simulink model "mcb_microchip_pmsm_autotuner_SAME70"  (R2023a)
settings: Solver=FixedStepDiscrete  StartTime=0.0  StopTime=30  RelTol=1e-3  EnableMultiTasking=on
InitFcn:
  | mcb_microchip_pmsm_autotuner_SAME70_data;
values from neighbouring files (symbols this model uses):
  PU_System = mcb_SetPUSystem(pmsm,inverter)    [mcb_microchip_pmsm_autotuner_SAME70_data.m]
  Ts = T_pwm    (= 5e-05)    [mcb_microchip_pmsm_autotuner_SAME70_data.m]
  Ts_motor = T_pwm/2    (= 2.5e-05)    [mcb_microchip_pmsm_autotuner_SAME70_data.m]
  Ts_simulink = T_pwm/2    (= 2.5e-05)    [mcb_microchip_pmsm_autotuner_SAME70_data.m]
  Ts_speed = 2 * Ts    (= 0.0001)    [mcb_microchip_pmsm_autotuner_SAME70_data.m]
undefined symbols (not defined in the file or in its folder): A24, AD10, AD7, inverter, LQFP144, MaxPer, ms, ns, PA0, PA1, PA10, PA11, PA12, PA13, PA16, PA18, PA9, PB0, PD18, PD19, PD24, PD25, PD26, PI_params, Pin, pmsm, Resol, SAME70Q21B, target, Timer, Unsigned
libraries: simulink x13, MCHP_Blockset x13, mcbcontrolslib x7, slpidlib x3, mcbpositiondecoderlib x3, svdutilitieslib x3, mcbplantlib x1, autolibpmsmexterior x1, focautotunershared x1
(part 4 of 4)

== system mcb_microchip_pmsm_autotuner_SAME70/Microcontroller/Input Scaling/Variant Subsystem/Automatic offset calibration ==
  Mode : Inport
  Iab_ADC : Inport  Port=2
  Add : Sum  Inputs=-+  RndMeth=Simplest  OutDataTypeStr=Inherit: Same as first input
  Compare To Constant : simulink/Logic and Bit Operations/Compare To Constant  relop=<  const=1  OutDataTypeStr=boolean
  Data Type Conversion : DataTypeConversion  OutDataTypeStr=int32  ConvertRealWorld=Stored Integer (SI)  RndMeth=Simplest  SaturateOnIntegerOverflow=off
  Enabled Subsystem : Subsystem  TreatAsAtomicUnit=on
  Gain : Gain  Gain=inverter.AmpPerCount  OutDataTypeStr=dataType  RndMeth=Simplest
  Iab : Outport
  wires:
  Data Type Conversion/1 -> Add/2, Enabled Subsystem/1(In1)
  Gain/1 -> Iab/1
  Enabled Subsystem/1(Out1) -> Add/1
  Add/1 -> Gain/1
  Compare To Constant/1 -> Enabled Subsystem/Enable
  Mode/1 -> Compare To Constant/1
  Iab_ADC/1 -> Data Type Conversion/1

== system mcb_microchip_pmsm_autotuner_SAME70/Microcontroller/Input Scaling/Variant Subsystem/Offser via parameter ==
  Mode : Inport
  Iab_ADC : Inport  Port=2
  Add : Sum  Inputs=-+  RndMeth=Simplest  OutDataTypeStr=Inherit: Same as first input
  Constant : Constant  Value=[inverter.CtSensAOffset inverter.CtSensBOffset]  OutDataTypeStr=Inherit: Inherit via back propagation
  Gain : Gain  Gain=inverter.AmpPerCount  OutDataTypeStr=dataType  RndMeth=Simplest
  Terminator : Terminator
  Iab : Outport
  wires:
  Gain/1 -> Iab/1
  Iab_ADC/1 -> Add/2
  Add/1 -> Gain/1
  Constant/1 -> Add/1
  Mode/1 -> Terminator/1

== system mcb_microchip_pmsm_autotuner_SAME70/Microcontroller/Output PWM Drivers/Sim/Subsystem ==
  PWM_In : Inport
  Constant : Constant  Value=0.5  OutDataTypeStr=dataType
  Gain : Gain  Gain=0.5  OutDataTypeStr=Inherit: Same as input
  Sum : Sum  Inputs=|++
  PWM_Duty_Cycles : Outport
  wires:
  Gain/1 -> Sum/1
  Constant/1 -> Sum/2
  PWM_In/1 -> Gain/1
  Sum/1 -> PWM_Duty_Cycles/1  "PWM_Duty_Cycles"

== system mcb_microchip_pmsm_autotuner_SAME70/Microcontroller/SCI In Abstraction/Variant Subsystem/Codegen ==
  SCI_Data : Inport
  Mode : Inport  Port=2
  AND : Logic  IconShape=distinctive  AllPortsSameDT=off  OutDataTypeStr=boolean
  Bus Creator : BusCreator  Inputs=4
  Compare To Constant : simulink/Logic and Bit Operations/Compare To Constant  relop=>=  const=2  OutDataTypeStr=boolean
  Data Type Conversion : DataTypeConversion  OutDataTypeStr=boolean  RndMeth=Simplest  SaturateOnIntegerOverflow=off
  Subsystem : Subsystem
  ConfigAndCommand : Outport
  DebugSel : Outport  Port=2
  wires:
  Bus Creator/1 -> ConfigAndCommand/1
  AND/1 -> Bus Creator/1  "Enable"
  Subsystem/1(Enable) -> AND/2
  Subsystem/2(AutoTuneEn) -> Data Type Conversion/1
  Subsystem/3(SpeedRef) -> Bus Creator/3  "SpeedRef"
  Subsystem/5(DebugSel) -> DebugSel/1
  Compare To Constant/1 -> AND/1
  Mode/1 -> Compare To Constant/1
  Subsystem/4(ResetPIParams) -> Bus Creator/4  "ResetPIGains"
  SCI_Data/1 -> Subsystem/1(SCI_Data)
  Data Type Conversion/1 -> Bus Creator/2  "AutoTuneEn"

== system mcb_microchip_pmsm_autotuner_SAME70/Microcontroller/SCI In Abstraction/Variant Subsystem/Sim ==
  SCI_Data : Inport
  Mode : Inport  Port=2
  AND : Logic  IconShape=distinctive  AllPortsSameDT=off  OutDataTypeStr=boolean
  Bus Creator : BusCreator  Inputs=4
  Compare To Constant : simulink/Logic and Bit Operations/Compare To Constant  relop=>=  const=2  OutDataTypeStr=boolean
  Constant : Constant  Value=1000  OutDataTypeStr=dataType  SampleTime=Ts
  Constant1 : Constant  OutDataTypeStr=uint8
  Constant2 : Constant  Value=0  OutDataTypeStr=boolean  SampleTime=Ts
  Data Type Conversion : DataTypeConversion  OutDataTypeStr=boolean  RndMeth=Simplest  SaturateOnIntegerOverflow=off
  Step : Step  Time=29  Before=1  After=0  SampleTime=Ts
  Step1 : Step  Time=4  SampleTime=Ts
  Terminator : Terminator
  ConfigAndCommand : Outport
  DebugSel : Outport  Port=2
  wires:
  SCI_Data/1 -> Terminator/1
  Mode/1 -> Compare To Constant/1
  Compare To Constant/1 -> AND/1
  Step/1 -> AND/2
  Bus Creator/1 -> ConfigAndCommand/1
  AND/1 -> Bus Creator/1  "Enable"
  Step1/1 -> Data Type Conversion/1
  Constant/1 -> Bus Creator/3  "SpeedRef"
  Constant1/1 -> DebugSel/1
  Constant2/1 -> Bus Creator/4  "ResetPIGains"
  Data Type Conversion/1 -> Bus Creator/2  "AutoTuneEn"

== system mcb_microchip_pmsm_autotuner_SAME70/Microcontroller/SCI_Rx/CodeGen/Subsystem ==
  In1 : Inport
  Enable1 : EnablePort
  Data : Outport
  wires:
  In1/1 -> Data/1

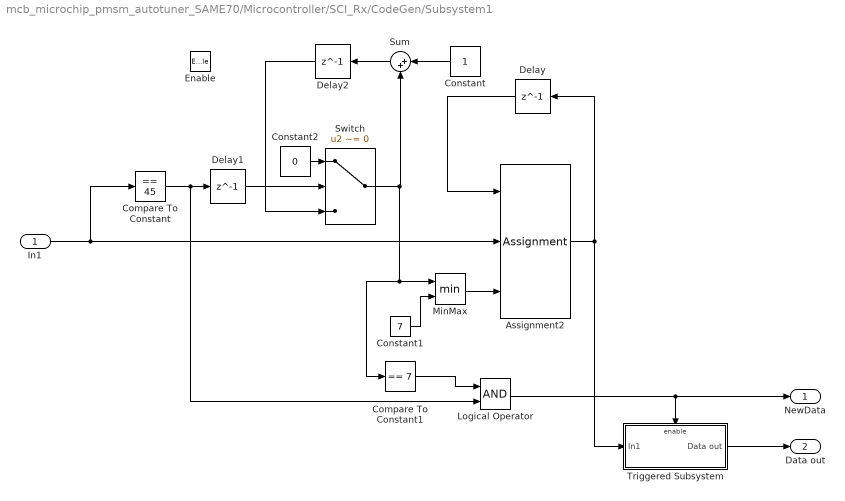
== system mcb_microchip_pmsm_autotuner_SAME70/Microcontroller/SCI_Rx/CodeGen/Subsystem1 ==
  In1 : Inport
  Enable : EnablePort
  Assignment2 : Assignment  IndexMode=Zero-based  DiagnosticForDimensions=Warning  IndexOptions=Starting index (port)  Indices=1  OutputSizes=1
  Compare To Constant : simulink/Logic and Bit Operations/Compare To Constant  relop===  const=45  OutDataTypeStr=boolean
  Compare To Constant1 : simulink/Logic and Bit Operations/Compare To Constant  relop===  const=7  OutDataTypeStr=boolean
  Constant : Constant  OutDataTypeStr=uint16  SampleTime=-1
  Constant1 : Constant  Value=7  OutDataTypeStr=uint16  SampleTime=-1
  Constant2 : Constant  Value=0  OutDataTypeStr=uint16  SampleTime=-1
  Delay : Delay  DelayLength=1  InitialCondition=[0 0 0 0 0 0 0 0]
  Delay1 : Delay  DelayLength=1  InitialCondition=0
  Delay2 : Delay  DelayLength=1  InitialCondition=0
  Logical Operator : Logic  AllPortsSameDT=off  OutDataTypeStr=boolean
  MinMax : MinMax  Inputs=2
  Sum : Sum  Inputs=|++
  Switch : Switch  Criteria=u2 ~= 0  SaturateOnIntegerOverflow=off  InputSameDT=off
  Triggered Subsystem : Subsystem  TreatAsAtomicUnit=on
  NewData : Outport  OutputWhenDisabled=reset  InitialOutput=0
  Data out : Outport  Port=2
  wires:
  Logical Operator/1 -> Triggered Subsystem/Enable, NewData/1
  Constant2/1 -> Switch/1
  Delay1/1 -> Switch/2
  Switch/1 -> MinMax/1, Compare To Constant1/1, Sum/2
  Sum/1 -> Delay2/1
  MinMax/1 -> Assignment2/3
  Constant1/1 -> MinMax/2
  Constant/1 -> Sum/1
  In1/1 -> Assignment2/2, Compare To Constant/1
  Compare To Constant1/1 -> Logical Operator/1
  Compare To Constant/1 -> Delay1/1, Logical Operator/2
  Delay2/1 -> Switch/3
  Delay/1 -> Assignment2/1
  Assignment2/1 -> Delay/1, Triggered Subsystem/1(In1)
  Triggered Subsystem/1(Data out) -> Data out/1

== system mcb_microchip_pmsm_autotuner_SAME70/Microcontroller/SCI_Tx/Codegen/Data ==
  Data : Inport
  Action Port : ActionPort  ActionPortLabel=else
  UART Tx : MCHP_Blockset/BUS UART/UART Tx  UART_REF=UART 0  ORDERING=None  AllOrNothing=off  SampleTime=-1  MCHP_MASTERLINK=mcb_microchip_pmsm_autotuner_SAME70/Microcontroller/Configurations/Microchip Master  NSend_Input=off  UART_String=off  NSend_Output=off
      settings: SourceProductName=MPLAB Device Blocks for Simulink
  wires:
  Data/1 -> UART Tx/1

== system mcb_microchip_pmsm_autotuner_SAME70/Microcontroller/SCI_Tx/Codegen/End ==
  Data : Inport
  Action Port : ActionPort  ActionPortLabel=elseif(u1 == single(target.SerialFrameSize-1))
  Mux : Mux  Inputs=2
  Start : Constant  Value=hex2dec('45')  OutDataTypeStr=uint8
  UART Tx : MCHP_Blockset/BUS UART/UART Tx  UART_REF=UART 0  ORDERING=None  AllOrNothing=off  SampleTime=-1  MCHP_MASTERLINK=mcb_microchip_pmsm_autotuner_SAME70/Microcontroller/Configurations/Microchip Master  NSend_Input=off  UART_String=off  NSend_Output=off
      settings: SourceProductName=MPLAB Device Blocks for Simulink
  wires:
  Start/1 -> Mux/2
  Data/1 -> Mux/1
  Mux/1 -> UART Tx/1

== system mcb_microchip_pmsm_autotuner_SAME70/Microcontroller/SCI_Tx/Codegen/Start ==
  Data : Inport
  Action Port : ActionPort  ActionPortLabel=if(u1 == 0)
  End : Constant  Value=hex2dec('53')  OutDataTypeStr=uint8
  Mux : Mux  Inputs=2
  UART Tx : MCHP_Blockset/BUS UART/UART Tx  UART_REF=UART 0  ORDERING=None  AllOrNothing=off  SampleTime=-1  MCHP_MASTERLINK=mcb_microchip_pmsm_autotuner_SAME70/Microcontroller/Configurations/Microchip Master  NSend_Input=off  UART_String=off  NSend_Output=off
      settings: SourceProductName=MPLAB Device Blocks for Simulink
  wires:
  End/1 -> Mux/1
  Data/1 -> Mux/2
  Mux/1 -> UART Tx/1

== system mcb_microchip_pmsm_autotuner_SAME70/Inverter and Motor/Inverter and Motor/Sim/Motor/Inverter ==
  Duty_abc : Inport
  Average-Value Inverter : mcbplantlib/Average-Value Inverter
  Constant2 : Constant  Value=inverter.V_dc  OutDataTypeStr=single  SampleTime=-1
  Data Type Conversion1 : DataTypeConversion  OutDataTypeStr=single  RndMeth=Simplest  SaturateOnIntegerOverflow=off
  Vabc : Outport
  wires:
  Constant2/1 -> Average-Value Inverter/2
  Duty_abc/1 -> Data Type Conversion1/1
  Average-Value Inverter/1 -> Vabc/1
  Data Type Conversion1/1 -> Average-Value Inverter/1

== system mcb_microchip_pmsm_autotuner_SAME70/Inverter and Motor/Inverter and Motor/Sim/Motor/Load_Profile (Torque) ==
  Data Type Conversion : DataTypeConversion  OutDataTypeStr=single  SaturateOnIntegerOverflow=off  RndMeth=Floor
  IIR Filter : mcbcontrolslib/IIR Filter  VariantControl=Low Pass Filter  VariantSelect=Low-pass  Filter_constant=0.0001  advancedSettings=off  Ts=50e-6  cutOff_freq=0.31834
  T_load : Step  Time=3  After=0  SampleTime=Ts_simulink
  Load_Trq : Outport  VectorParamsAs1DForOutWhenUnconnected=off
  wires:
  Data Type Conversion/1 -> IIR Filter/1
  IIR Filter/1 -> Load_Trq/1
  T_load/1 -> Data Type Conversion/1

== system mcb_microchip_pmsm_autotuner_SAME70/Microcontroller/Application/Current Control/Current_Controllers/PI_Controller_Id ==
  I_ref : Inport
  I_fb : Inport  Port=2
  En : Inport  Port=3
  PIParams : Inport  Port=4
  Bus Selector : BusSelector  OutputSignals=KpId,KiId
  Discrete PI Controller with anti-windup & reset : slpidlib/PID Controller  Controller=PI  Form=Parallel  TimeDomain=Discrete-time  UseExternalTs=off  SampleTime=-1  IntegratorMethod=Forward Euler  FilterMethod=Forward Euler  ControllerParametersSource=external  P=1  I=1  UseKiTs=on  D=0  N=100  UseFilter=on  TunerSelectOption=Transfer Function Based (PID Tuner App)  InitialConditionSource=external  InitialConditionForIntegrator=0  InitialConditionForFilter=0  DifferentiatorICPrevScaledInput=0  ExternalReset=level  TrackingMode=off  Kt=1  LimitOutput=on  SatLimitsSource=internal  UpperSaturationLimit=1  LowerSaturationLimit=-1  LinearizeAsGain=on  AntiWindupMode=clamping  Kb=1  LimitIntegrator=off  UpperIntegratorSaturationLimit=inf  LowerIntegratorSaturationLimit=-inf  RndMeth=Simplest  POutMin=[]  POutMax=[]  IOutMin=[]  IOutMax=[]  DOutMin=[]  DOutMax=[]  NOutMin=[]  NOutMax=[]  SumOutMin=[]  SumOutMax=[]  SaturationOutDataTypeStr=Inherit: Inherit via back propagation  SaturationOutMin=[]  SaturationOutMax=[]  PParamMin=[]  PParamMax=[]  IParamMin=[]  IParamMax=[]  DParamMin=[]  DParamMax=[]  NParamMin=[]  NParamMax=[]  KbParamMin=[]  KbParamMax=[]  KtParamMin=[]  KtParamMax=[]  KbOutMin=[]  KbOutMax=[]  KtOutMin=[]  KtOutMax=[]  IntegratorOutMin=[]  IntegratorOutMax=[]  FilterOutMin=[]  FilterOutMax=[]  SumI1OutMin=[]  SumI1OutMax=[]  SumI2OutMin=[]  SumI2OutMax=[]  SumI3OutMin=[]  SumI3OutMax=[]  SumI4OutMin=[]  SumI4OutMax=[]  SumDOutMin=[]  SumDOutMax=[]  DifferentiatorOutMin=[]  DifferentiatorOutMax=[]  FilterDiffOutCoefMin=[]  FilterDiffOutCoefMax=[]  ReciprocalOutMin=[]  ReciprocalOutMax=[]  SumDenOutMin=[]  SumDenOutMax=[]  SumNumOutMin=[]  SumNumOutMax=[]  DivideOutMin=[]  DivideOutMax=[]  UdiffTsProdOutMin=[]  UdiffTsProdOutMax=[]  NTsProdOutMin=[]  NTsProdOutMax=[]  UintegralTsProdOutMin=[]  UintegralTsProdOutMax=[]  UngainTsProdOutMin=[]  UngainTsProdOutMax=[]  ClampingZeroOutDataTypeStr=Inherit: Inherit via back propagation  ClampingZeroOutMin=[]  ClampingZeroOutMax=[]  FilterDenConstantOutDataTypeStr=Inherit: Inherit via back propagation  FilterDenConstantOutMin=[]  FilterDenConstantOutMax=[]  PCopyOutDataTypeStr=Inherit: Inherit via back propagation  PCopyOutMin=[]  PCopyOutMax=[]  NCopyOutDataTypeStr=Inherit: Inherit via back propagation  NCopyOutMin=[]  NCopyOutMax=[]  IntegratorContinuousStateAttributes=''  IntegratorStateMustResolveToSignalObject=off  IntegratorRTWStateStorageClass=Auto  FilterContinuousStateAttributes=''  FilterStateMustResolveToSignalObject=off  FilterRTWStateStorageClass=Auto  ParallelPVariant=ExternalParameters  IdealPVariant=Disabled  IVariant=ExternalParameters  DVariant=Disabled  IntegratorVariant=Discrete  SatVariant=Enabled  AWVariant=DiscClampingParallel  PCopyVariant=Disabled  TRVariant=Disabled  FdbkBlocksVariant=Forward  IdealPFdbkVariant=Disabled  SatFdbkVariant=Disabled  DerivativeFilterVariant=Disabled  NVariant=Disabled  NCopyVariant=Disabled_SignalSpec  FilterICVariant=Disabled  IntegratorICVariant=ExternalICs  ExternalResetVariant=ExternalReset  TRSumVariant=Passthrough  SumFdbkVariant=Disabled  SumVariant=Sum_PI  TsampFilterVariant=InternalTs  TsampNgainVariant=Passthrough  TsampIntegralVariant=Disabled_SignalSpec  ExternalSaturationOutDataTypeStr=Inherit: Same as second input
  Gain : Gain  Gain=Ts
  Logical Operator : Logic  Operator=NOT  IconShape=distinctive  AllPortsSameDT=off  OutDataTypeStr=boolean
  Sum : Sum  Inputs=|+-  OutDataTypeStr=Inherit: Same as first input
  Switch : Switch  Criteria=u2 ~= 0  RndMeth=Simplest  SaturateOnIntegerOverflow=off  InputSameDT=off
  Unit Delay : UnitDelay  SampleTime=-1  HasFrameUpgradeWarning=on
  Vd_OpenLoop : Constant  Value=0.1  OutDataTypeStr=dataType  SampleTime=-1
  V_ref : Outport  VectorParamsAs1DForOutWhenUnconnected=off
  wires:
  Switch/1 -> V_ref/1, Unit Delay/1
  I_fb/1 -> Sum/2
  Sum/1 -> Discrete PI Controller with anti-windup & reset/1
  I_ref/1 -> Sum/1
  Logical Operator/1 -> Discrete PI Controller with anti-windup & reset/4
  Unit Delay/1 -> Discrete PI Controller with anti-windup & reset/5
  Discrete PI Controller with anti-windup & reset/1 -> Switch/1
  En/1 -> Logical Operator/1, Switch/2
  Vd_OpenLoop/1 -> Switch/3
  Bus Selector/2 -> Gain/1  "<KiId>"
  Bus Selector/1 -> Discrete PI Controller with anti-windup & reset/2  "<KpId>"
  Gain/1 -> Discrete PI Controller with anti-windup & reset/3
  PIParams/1 -> Bus Selector/1

== system mcb_microchip_pmsm_autotuner_SAME70/Microcontroller/Application/Current Control/Current_Controllers/PI_Controller_Iq ==
  I_ref : Inport
  I_fb : Inport  Port=2
  En : Inport  Port=3
  PIParams : Inport  Port=4
  Bus Selector : BusSelector  OutputSignals=KpIq,KiIq
  Discrete PI Controller with anti-windup & reset : slpidlib/PID Controller  Controller=PI  Form=Parallel  TimeDomain=Discrete-time  UseExternalTs=off  SampleTime=-1  IntegratorMethod=Forward Euler  FilterMethod=Forward Euler  ControllerParametersSource=external  P=1  I=1  UseKiTs=on  D=0  N=100  UseFilter=on  TunerSelectOption=Transfer Function Based (PID Tuner App)  InitialConditionSource=external  InitialConditionForIntegrator=0  InitialConditionForFilter=0  DifferentiatorICPrevScaledInput=0  ExternalReset=level  TrackingMode=off  Kt=1  LimitOutput=on  SatLimitsSource=internal  UpperSaturationLimit=1  LowerSaturationLimit=-1  LinearizeAsGain=on  AntiWindupMode=clamping  Kb=1  LimitIntegrator=off  UpperIntegratorSaturationLimit=inf  LowerIntegratorSaturationLimit=-inf  RndMeth=Simplest  POutMin=[]  POutMax=[]  IOutMin=[]  IOutMax=[]  DOutMin=[]  DOutMax=[]  NOutMin=[]  NOutMax=[]  SumOutMin=[]  SumOutMax=[]  SaturationOutDataTypeStr=Inherit: Inherit via back propagation  SaturationOutMin=[]  SaturationOutMax=[]  PParamMin=[]  PParamMax=[]  IParamMin=[]  IParamMax=[]  DParamMin=[]  DParamMax=[]  NParamMin=[]  NParamMax=[]  KbParamMin=[]  KbParamMax=[]  KtParamMin=[]  KtParamMax=[]  KbOutMin=[]  KbOutMax=[]  KtOutMin=[]  KtOutMax=[]  IntegratorOutMin=[]  IntegratorOutMax=[]  FilterOutMin=[]  FilterOutMax=[]  SumI1OutMin=[]  SumI1OutMax=[]  SumI2OutMin=[]  SumI2OutMax=[]  SumI3OutMin=[]  SumI3OutMax=[]  SumI4OutMin=[]  SumI4OutMax=[]  SumDOutMin=[]  SumDOutMax=[]  DifferentiatorOutMin=[]  DifferentiatorOutMax=[]  FilterDiffOutCoefMin=[]  FilterDiffOutCoefMax=[]  ReciprocalOutMin=[]  ReciprocalOutMax=[]  SumDenOutMin=[]  SumDenOutMax=[]  SumNumOutMin=[]  SumNumOutMax=[]  DivideOutMin=[]  DivideOutMax=[]  UdiffTsProdOutMin=[]  UdiffTsProdOutMax=[]  NTsProdOutMin=[]  NTsProdOutMax=[]  UintegralTsProdOutMin=[]  UintegralTsProdOutMax=[]  UngainTsProdOutMin=[]  UngainTsProdOutMax=[]  ClampingZeroOutDataTypeStr=Inherit: Inherit via back propagation  ClampingZeroOutMin=[]  ClampingZeroOutMax=[]  FilterDenConstantOutDataTypeStr=Inherit: Inherit via back propagation  FilterDenConstantOutMin=[]  FilterDenConstantOutMax=[]  PCopyOutDataTypeStr=Inherit: Inherit via back propagation  PCopyOutMin=[]  PCopyOutMax=[]  NCopyOutDataTypeStr=Inherit: Inherit via back propagation  NCopyOutMin=[]  NCopyOutMax=[]  IntegratorContinuousStateAttributes=''  IntegratorStateMustResolveToSignalObject=off  IntegratorRTWStateStorageClass=Auto  FilterContinuousStateAttributes=''  FilterStateMustResolveToSignalObject=off  FilterRTWStateStorageClass=Auto  ParallelPVariant=ExternalParameters  IdealPVariant=Disabled  IVariant=ExternalParameters  DVariant=Disabled  IntegratorVariant=Discrete  SatVariant=Enabled  AWVariant=DiscClampingParallel  PCopyVariant=Disabled  TRVariant=Disabled  FdbkBlocksVariant=Forward  IdealPFdbkVariant=Disabled  SatFdbkVariant=Disabled  DerivativeFilterVariant=Disabled  NVariant=Disabled  NCopyVariant=Disabled_SignalSpec  FilterICVariant=Disabled  IntegratorICVariant=ExternalICs  ExternalResetVariant=ExternalReset  TRSumVariant=Passthrough  SumFdbkVariant=Disabled  SumVariant=Sum_PI  TsampFilterVariant=InternalTs  TsampNgainVariant=Passthrough  TsampIntegralVariant=Disabled_SignalSpec  ExternalSaturationOutDataTypeStr=Inherit: Same as second input
  Gain : Gain  Gain=Ts
  Logical Operator : Logic  Operator=NOT  IconShape=distinctive  AllPortsSameDT=off  OutDataTypeStr=boolean
  Sum : Sum  Inputs=|+-  OutDataTypeStr=Inherit: Same as first input
  Switch : Switch  Criteria=u2 ~= 0  RndMeth=Simplest  SaturateOnIntegerOverflow=off  InputSameDT=off
  Unit Delay : UnitDelay  SampleTime=-1  HasFrameUpgradeWarning=on
  Vq_OpenLoop : Constant  Value=0  OutDataTypeStr=dataType  SampleTime=-1
  V_ref : Outport  VectorParamsAs1DForOutWhenUnconnected=off
  wires:
  Switch/1 -> V_ref/1, Unit Delay/1
  I_fb/1 -> Sum/2
  Sum/1 -> Discrete PI Controller with anti-windup & reset/1
  I_ref/1 -> Sum/1
  Logical Operator/1 -> Discrete PI Controller with anti-windup & reset/4
  Unit Delay/1 -> Discrete PI Controller with anti-windup & reset/5
  Discrete PI Controller with anti-windup & reset/1 -> Switch/1
  Vq_OpenLoop/1 -> Switch/3
  En/1 -> Logical Operator/1, Switch/2
  Bus Selector/2 -> Gain/1  "<KiIq>"
  Bus Selector/1 -> Discrete PI Controller with anti-windup & reset/2  "<KpIq>"
  Gain/1 -> Discrete PI Controller with anti-windup & reset/3
  PIParams/1 -> Bus Selector/1

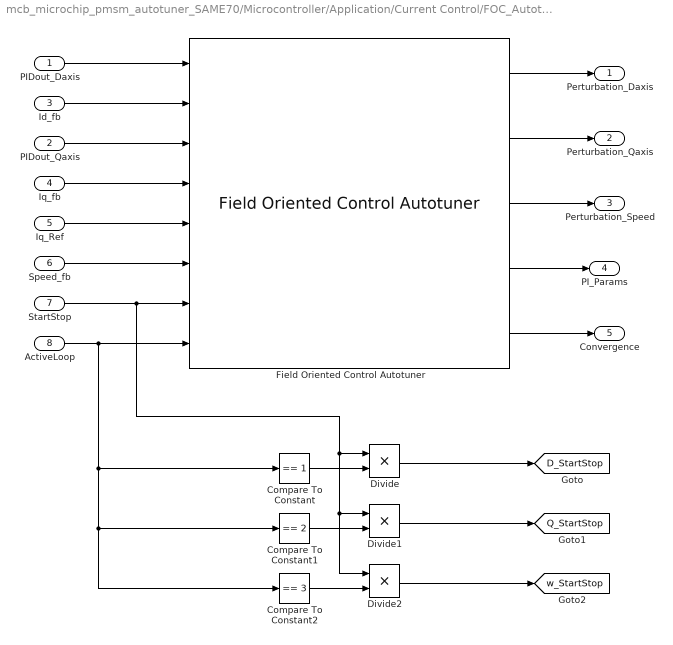
== system mcb_microchip_pmsm_autotuner_SAME70/Microcontroller/Application/Current Control/FOC_Autotuner/FOC_Autotuner ==
  PIDout_Daxis : Inport
  PIDout_Qaxis : Inport  Port=2
  Id_fb : Inport  Port=3
  Iq_fb : Inport  Port=4
  Iq_Ref : Inport  Port=5
  Speed_fb : Inport  Port=6
  StartStop : Inport  Port=7
  ActiveLoop : Inport  Port=8
  Compare To Constant : simulink/Logic and Bit Operations/Compare To Constant  relop===  const=1  OutDataTypeStr=boolean
  Compare To Constant1 : simulink/Logic and Bit Operations/Compare To Constant  relop===  const=2  OutDataTypeStr=boolean
  Compare To Constant2 : simulink/Logic and Bit Operations/Compare To Constant  relop===  const=3  OutDataTypeStr=boolean
  Divide : Product  Inputs=**
  Divide1 : Product  Inputs=**
  Divide2 : Product  Inputs=**
  Field Oriented Control Autotuner : focautotunershared/Field Oriented Control Autotuner  TuneDaxisLoop=on  TuneQaxisLoop=on  TuneSpeedLoop=on  TuneFluxLoop=off  UseSameSettingsInner=on  UseSameSettingsOuter=off  TsExperiment=-1  TimeDomain=discrete-time  TsTuning=Ts_tuning  UseTuningTs=on  PIDTypeAllInner=PI  PIDFormAllInner=Parallel  TsAllInner=Ts  IntegratorMethodAllInner=Forward Euler  FilterMethodAllInner=Forward Euler  BandwidthAllInner=PI_params.CurrentBW  TargetPMAllInner=PI_params.CurrentPhaseMargin  PIDTypeDaxis=PI  PIDFormDaxis=Parallel  TsDaxis=Ts  IntegratorMethodDaxis=Forward Euler  FilterMethodDaxis=Forward Euler  BandwidthDaxis=PI_params.CurrentBW  TargetPMDaxis=PI_params.CurrentPhaseMargin  PIDTypeQaxis=PI  PIDFormQaxis=Parallel  TsQaxis=Ts  IntegratorMethodQaxis=Forward Euler  FilterMethodQaxis=Forward Euler  BandwidthQaxis=PI_params.CurrentBW  TargetPMQaxis=PI_params.CurrentPhaseMargin  PIDTypeAllOuter=PI  PIDFormAllOuter=Parallel  TsAllOuter=0.1  IntegratorMethodAllOuter=Forward Euler  FilterMethodAllOuter=Forward Euler  BandwidthAllOuter=1  TargetPMAllOuter=60  PIDTypeSpeed=PI  PIDFormSpeed=Parallel  TsSpeed=Ts_speed  IntegratorMethodSpeed=Forward Euler  FilterMethodSpeed=Forward Euler  BandwidthSpeed=PI_params.SpeedBW  TargetPMSpeed=PI_params.SpeedPhaseMargin  PIDTypeFlux=PI  PIDFormFlux=Parallel  TsFlux=0.1  IntegratorMethodFlux=Forward Euler  FilterMethodFlux=Forward Euler  BandwidthFlux=1  TargetPMFlux=60  StartTimeDaxis=1  DurationDaxis=0.05  StopTimeDaxis=1.05  StartTimeQaxis=1.1  DurationQaxis=0.05  StopTimeQaxis=1.15  StartTimeSpeed=2  DurationSpeed=3  StopTimeSpeed=5  StartTimeFlux=6  DurationFlux=3  StopTimeFlux=9  ExperimentMode=Sinestream  PlantTypeAllInner=Stable  PlantSignAllInner=Positive  AmpSineAllInner=PI_params.CurrentSineAmp  PlantTypeDaxis=Stable  PlantSignDaxis=Positive  AmpSineDaxis=PI_params.CurrentSineAmp  PlantTypeQaxis=Stable  PlantSignQaxis=Positive  AmpSineQaxis=PI_params.CurrentSineAmp  PlantTypeAllOuter=Stable  PlantSignAllOuter=Positive  AmpSineAllOuter=1  PlantTypeSpeed=Stable  PlantSignSpeed=Positive  AmpSineSpeed=PI_params.SpeedSineAmp  PlantTypeFlux=Stable  PlantSignFlux=Positive  AmpSineFlux=1  UseExternalWc=off  UseExternalPM=off  UseExternalSourceStartStop=on  UseExternalAmpSine=off  UseExternalAchievedPM=off  UseExternalFRD=off  UseExternalU0=off  UseExternalActiveLoop=off  BlockDataType=single  variantStartStop=variantExternal  variantBandwidth=variantInternal  variantPhaseMargin=variantInternal  variantSineAmplitudes=variantInternal  variantEnableDaxis=variantLoopEnabled  variantEnableQaxis=variantLoopEnabled  variantEnableSpeed=variantLoopEnabled  variantEnableFlux=variantLoopDisabled  variantBandwidthDaxis=variantExternal  variantBandwidthQaxis=variantExternal  variantBandwidthSpeed=variantExternal  variantBandwidthFlux=variantExternal  variantSingleMultiRate=DifferentSamplingRates  variantValidDaxisSampleTime=variantValidTs  variantValidQaxisSampleTime=variantValidTs  variantValidSpeedSampleTime=variantValidTs  variantValidFluxSampleTime=variantValidTs  focMode=focMode  EstimationWindowSize=3
  Perturbation_Daxis : Outport
  Perturbation_Qaxis : Outport  Port=2
  Perturbation_Speed : Outport  Port=3
  PI_Params : Outport  Port=4
  Convergence : Outport  Port=5
  tag scope: D_StartStop=global, Q_StartStop=global, w_StartStop=global
  wires:
  Divide2/1 -> [w_StartStop]
  Compare To Constant2/1 -> Divide2/2
  Divide1/1 -> [Q_StartStop]
  Compare To Constant1/1 -> Divide1/2
  Divide/1 -> [D_StartStop]
  Compare To Constant/1 -> Divide/2
  ActiveLoop/1 -> Compare To Constant/1, Compare To Constant1/1, Compare To Constant2/1, Field Oriented Control Autotuner/8
  StartStop/1 -> Divide/1, Divide1/1, Divide2/1, Field Oriented Control Autotuner/7
  Field Oriented Control Autotuner/3 -> Perturbation_Speed/1
  Field Oriented Control Autotuner/1 -> Perturbation_Daxis/1
  Field Oriented Control Autotuner/4 -> PI_Params/1
  Field Oriented Control Autotuner/2 -> Perturbation_Qaxis/1
  Field Oriented Control Autotuner/5 -> Convergence/1
  Iq_fb/1 -> Field Oriented Control Autotuner/4
  Speed_fb/1 -> Field Oriented Control Autotuner/6
  PIDout_Qaxis/1 -> Field Oriented Control Autotuner/3
  Id_fb/1 -> Field Oriented Control Autotuner/2
  PIDout_Daxis/1 -> Field Oriented Control Autotuner/1
  Iq_Ref/1 -> Field Oriented Control Autotuner/5

== system mcb_microchip_pmsm_autotuner_SAME70/Microcontroller/Application Abstraction/Variant Subsystem/Index Absent/Enabled Subsystem ==
  In1 : Inport
  Enable : EnablePort
  Out1 : Outport
  wires:
  In1/1 -> Out1/1

== system mcb_microchip_pmsm_autotuner_SAME70/Microcontroller/Input HW Drivers/Codegen/Qdec_interface/If Action Subsystem ==
  In1 : Inport
  Action Port : ActionPort  ActionPortLabel=if((u1 > 49151 ) & (u2 < 16384 ))
  Add : Sum
  Constant : Constant  Value=(EnCountPerRev) -mod(65536,(EnCountPerRev))  OutDataTypeStr=uint16
  Out1 : Outport
  wires:
  In1/1 -> Add/1
  Constant/1 -> Add/2
  Add/1 -> Out1/1

== system mcb_microchip_pmsm_autotuner_SAME70/Microcontroller/Input HW Drivers/Codegen/Qdec_interface/If Action Subsystem1 ==
  In1 : Inport
  Action Port : ActionPort  ActionPortLabel=elseif((u2 > 49151 ) & (u1 < 16384 ))
  Add : Sum
  Constant : Constant  Value=mod(65536,(EnCountPerRev))  OutDataTypeStr=uint16
  Out1 : Outport
  wires:
  Add/1 -> Out1/1
  Constant/1 -> Add/2
  In1/1 -> Add/1

== system mcb_microchip_pmsm_autotuner_SAME70/Microcontroller/Input HW Drivers/Codegen/Qdec_interface/If Action Subsystem2 ==
  In1 : Inport
  Action Port : ActionPort  ActionPortLabel=else
  Out1 : Outport
  wires:
  In1/1 -> Out1/1

== system mcb_microchip_pmsm_autotuner_SAME70/Microcontroller/Input HW Drivers/Codegen/Qdec_interface/Offset ==
  QdecCount : Inport
  Enable : EnablePort
  Add1 : Sum  Inputs=-+  OutDataTypeStr=uint16
  Constant2 : Constant  Value=EnCountPerRev  OutDataTypeStr=Inherit: Inherit via back propagation
  Data Store Write : DataStoreWrite  DataStoreName=PosOffset  IndexOptions=Index vector (dialog)  Indices=1  OutputSizes=1
  Math Function1 : Math  Operator=mod  SignedPower=on
  wires:
  QdecCount/1 -> Math Function1/1
  Constant2/1 -> Add1/2, Math Function1/2
  Add1/1 -> Data Store Write/1
  Math Function1/1 -> Add1/1

== system mcb_microchip_pmsm_autotuner_SAME70/Microcontroller/Input Scaling/Variant Subsystem/Automatic offset calibration/Enabled Subsystem ==
  In1 : Inport
  Enable : EnablePort
  Out1 : Outport
  wires:
  In1/1 -> Out1/1

== system mcb_microchip_pmsm_autotuner_SAME70/Microcontroller/SCI In Abstraction/Variant Subsystem/Codegen/Subsystem ==
  SCI_Data : Inport
  Bitwise OR : simulink/Logic and Bit Operations/Bitwise Operator  logicop=OR  UseBitMask=off  NumInputPorts=2  BitMask=bin2dec('11011001')  BitMaskRealWorld=Stored Integer
      settings: LibrarySourceBlock=|
      | simulink/Quick Insert/Logic and Bit
      | Operations/Bitwise OR
  Data Type Conversion : DataTypeConversion  OutDataTypeStr=uint16  RndMeth=Simplest  SaturateOnIntegerOverflow=off
  Data Type Conversion1 : DataTypeConversion  OutDataTypeStr=uint16  RndMeth=Simplest  SaturateOnIntegerOverflow=off
  Data Type Conversion2 : DataTypeConversion  OutDataTypeStr=int16  ConvertRealWorld=Stored Integer (SI)  RndMeth=Simplest  SaturateOnIntegerOverflow=off
  Data Type Conversion3 : DataTypeConversion  OutDataTypeStr=dataType  RndMeth=Simplest  SaturateOnIntegerOverflow=off
  Demux : Demux  Outputs=8
  Shift Arithmetic : ArithShift  BitShiftNumber=8  BitShiftDirection=Left
  Terminator1 : Terminator
  Terminator2 : Terminator
  Enable : Outport
  AutoTuneEn : Outport  Port=2
  SpeedRef : Outport  Port=3
  ResetPIParams : Outport  Port=4
  DebugSel : Outport  Port=5
  wires:
  SCI_Data/1 -> Demux/1
  Demux/1 -> Data Type Conversion/1
  Demux/2 -> Data Type Conversion1/1
  Data Type Conversion/1 -> Bitwise OR/1
  Data Type Conversion1/1 -> Shift Arithmetic/1
  Shift Arithmetic/1 -> Bitwise OR/2
  Bitwise OR/1 -> Data Type Conversion2/1
  Demux/3 -> Enable/1
  Demux/4 -> AutoTuneEn/1
  Demux/6 -> DebugSel/1
  Demux/7 -> Terminator2/1
  Data Type Conversion2/1 -> Data Type Conversion3/1
  Demux/5 -> ResetPIParams/1
  Data Type Conversion3/1 -> SpeedRef/1
  Demux/8 -> Terminator1/1

== system mcb_microchip_pmsm_autotuner_SAME70/Microcontroller/SCI_Rx/CodeGen/Subsystem1/Triggered Subsystem ==
  In1 : Inport
  Enable : EnablePort
  Data out : Outport
  wires:
  In1/1 -> Data out/1

== stateflow chart mcb_microchip_pmsm_autotuner_SAME70/Microcontroller/Application/Autotuner Mode Control/Chart ==
  state Run1
    state Tuning
      state EndOftuning
        entry: ActiveLoop = 0;
        KpSpeed = KpSpeedAT;
        KiSpeed = KiSpeedAT;
        during: tuningInProgress = 0;
      state Inactive
        entry: tuningInProgress = 1;
        during: StartStop = 0;
      state DaxisLoop
        entry: ActiveLoop = 1;
        during: StartStop = 1;
      state Tuning
        during: StartStop = 0;
      state SpeedLoop
        entry: ActiveLoop = 3;
        KpIq = KpIqAT;
        KiIq = KiIqAT;
        during: StartStop = 1;
      state QaxisLoop
        entry: ActiveLoop = 2;
        KpId = KpIdAT;
        KiId = KiIdAT;
        during: StartStop = 1;
      (default) -> Inactive
      Run1.Tuning.Tuning -> EndOftuning [order 3] : after(1,sec)[ActiveLoop == 3]
      Inactive -> DaxisLoop : after(0.5, sec)
      DaxisLoop -> Run1.Tuning.Tuning : after(1, sec)
      SpeedLoop -> Run1.Tuning.Tuning : after(11, sec)
      Run1.Tuning.Tuning -> QaxisLoop [order 1] : after(1,sec)[ActiveLoop == 1]
      QaxisLoop -> Run1.Tuning.Tuning : after(1, sec)
      Run1.Tuning.Tuning -> SpeedLoop [order 2] : after(1,sec)[ActiveLoop == 2]
    state NotTuning
      entry:
      PIParamsUpdated = false;
      during: tuningInProgress = 0;
    state ResetPI
      entry:
      KpId = KpIdDef;
      KiId = KiIdDef;
      KpIq = KpIqDef;
      KiIq = KiIqDef;
      KpSpeed = KpSpeedDef;
      KiSpeed = KiSpeedDef;
      PIParamsUpdated = true;
    (default) -> NotTuning
    Run1.Tuning -> NotTuning : [tune == 0 && tuningInProgress != 1]
    NotTuning -> Run1.Tuning [order 1] : [tune == 1 && tuningInProgress != 1]
    NotTuning -> ResetPI [order 2] : [ResetPI == true && ResetPIPrev == false]
    ResetPI -> NotTuning : [PIParamsUpdated == true]
  state Init
    entry:
    KpId = KpIdDef;
    KiId = KiIdDef;
    KpIq = KpIqDef;
    KiIq = KiIqDef;
    KpSpeed = KpSpeedDef;
    KiSpeed = KiSpeedDef;
  (default) -> Init
  Init -> Run1 : [Enable == true]
  data: tune input boolean; tuningInProgress local boolean; ActiveLoop output uint16; StartStop output boolean; ResetPI input; ResetPIPrev input; PIParamsUpdated local double; KiIdAT input; KiIdDef input; KiIqAT input; KiIqDef input; KiSpeedAT input; KiSpeedDef input; KpIdAT input; KpIdDef input; KpIqAT input; KpIqDef input; KpSpeedAT input; KpSpeedDef input; KiId output double; KiIq output double; KiSpeed output double; KpId output double; KpIq output double; KpSpeed output double; Enable input
